simulink model "Sensors"  (R2016b)
settings: Solver=ode45  StartTime=0.0  StopTime=10.0  RelTol=1e-3  EnableMultiTasking=on
undefined symbols (not defined in the file): Amc_flgAirMassFlowOverride, Amc_uSensMaxValid, Amc_uSensMinValid, Bvc_rVoltDivHigh, Bvc_rVoltDivLow, Bvc_uBattMax, Bvc_uBattMin, Cpc_flgPChargeOverride, Ctc_rPullUp_C, Ctc_uSensMaxValid, Ctc_uSensMinValid, Ctc_uSupply, Egc_facEgasMan, Egc_flgEgasOverride, Egc_stEgasFilt, Egc_tiTEgasFilt, Egc_uSensMaxValid, Egc_uSensMinValid, Mpc_uSensMaxValid, Mpc_uSensMinValid, Mtc_rPullUp_C, Mtc_uSensMaxValid, Mtc_uSensMinValid, Mtc_uSupply, Opc_rpmEngMinOilPressure
libraries: simulink x8
(part 2 of 2)

== system Sensors/Sensors_mdl/Opc/G1_Digital_Input_Receive ==
  Data Type Conversion2 : DataTypeConversion  OutMin=0.0  OutMax=1.0  OutDataTypeStr=boolean
  Data Type Conversion3 : DataTypeConversion  OutMin=0.0  OutMax=1.0  OutDataTypeStr=boolean
  FlexECU_DevLib_FcnAPI_Wrapper_SFcn : S-Function  FunctionName=ehooks_medc17flex_devlib_basic_io_fcncall  Parameters=NoInputPorts, NoOutputPorts, InputPortDataTypes, OutputPortDataTypes, CFunctionArgTypes, CFunctionName, ChannelName  SFunctionDeploymentMode=off  EnableBusSupport=off  mask{NoInputPorts=0, NoOutputPorts=2, InputPortDataTypes=, OutputPortDataTypes=uint8,uint8, CFunctionArgTypes=ret,ref, CFunctionName=DevLib_Dio_Get, ChannelName=I_S_DIG13}
      mask prompts: NoInputPorts "Number of input ports"; NoOutputPorts "Number of output ports"; InputPortDataTypes "Input port data types"; OutputPortDataTypes "Output port data types"; CFunctionArgTypes "C function argument types"; CFunctionName "C function name"; ChannelName "Channel (pin) name"
      mask Display: disp('EHOOKS FlexECU\nDevLib Wrapper\nS-Function')
  status : Outport
  stRaw1 : Outport  Port=2
  wires:
  FlexECU_DevLib_FcnAPI_Wrapper_SFcn/2 -> Data Type Conversion2/1
  FlexECU_DevLib_FcnAPI_Wrapper_SFcn/1 -> Data Type Conversion3/1
  Data Type Conversion3/1 -> status/1
  Data Type Conversion2/1 -> stRaw1/1

== system Sensors/Sensors_mdl/Cpc/Cpc_calc/Accumulator ==
  in : Inport
  initValue : Inport  Port=2
  Add : Sum
  MATLAB Function : MATLAB Function  TreatAsAtomicUnit=on
  Switch2 : Switch  Threshold=1
  Unit Delay : UnitDelay  SampleTime=-1
  Out2 : Outport
  wires:
  in/1 -> Add/1, MATLAB Function/1(u)
  Unit Delay/1 -> Add/2
  Switch2/1 -> Out2/1
  initValue/1 -> Switch2/3
  Add/1 -> Switch2/1, Unit Delay/1
  MATLAB Function/1(y) -> Switch2/2

== system Sensors/Sensors_mdl/Cpc/Cpc_calc/Counter ==
  in : Inport
  Add1 : Sum
  Constant1 : Constant  OutDataTypeStr=single
  Constant2 : Constant  Value=0  OutDataTypeStr=single
  MATLAB Function : MATLAB Function  TreatAsAtomicUnit=on
  Switch2 : Switch  Threshold=1
  Unit Delay1 : UnitDelay  SampleTime=-1
  Out1 : Outport
  wires:
  Constant1/1 -> Add1/1
  Unit Delay1/1 -> Add1/2
  Switch2/1 -> Out1/1
  Constant2/1 -> Switch2/3
  Add1/1 -> Switch2/1, Unit Delay1/1
  MATLAB Function/1(y) -> Switch2/2
  in/1 -> MATLAB Function/1(u)

== system Sensors/Sensors_mdl/Cpc/Cpc_get/G1_ADC_Input_Receive ==
  Data Type Conversion2 : DataTypeConversion  OutMin=0.0  OutMax=5.0  OutDataTypeStr=single
  Data Type Conversion3 : DataTypeConversion  OutMin=0.0  OutMax=1.0  OutDataTypeStr=boolean
  FlexECU_DevLib_FcnAPI_Wrapper_SFcn : S-Function  FunctionName=ehooks_medc17flex_devlib_basic_io_fcncall  Parameters=NoInputPorts, NoOutputPorts, InputPortDataTypes, OutputPortDataTypes, CFunctionArgTypes, CFunctionName, ChannelName  SFunctionDeploymentMode=off  EnableBusSupport=off  mask{NoInputPorts=0, NoOutputPorts=2, InputPortDataTypes=, OutputPortDataTypes=uint8,int16, CFunctionArgTypes=ret,ref, CFunctionName=DevLib_Adc_Get, ChannelName=I_A_AN05}
      mask prompts: NoInputPorts "Number of input ports"; NoOutputPorts "Number of output ports"; InputPortDataTypes "Input port data types"; OutputPortDataTypes "Output port data types"; CFunctionArgTypes "C function argument types"; CFunctionName "C function name"; ChannelName "Channel (pin) name"
      mask Display: disp('EHOOKS FlexECU\nDevLib Wrapper\nS-Function')
  Gain : Gain  Gain=5/1023  OutDataTypeStr=Inherit: Same as input
  status : Outport
  uRaw : Outport  Port=2
  wires:
  FlexECU_DevLib_FcnAPI_Wrapper_SFcn/1 -> Data Type Conversion3/1
  FlexECU_DevLib_FcnAPI_Wrapper_SFcn/2 -> Data Type Conversion2/1
  Gain/1 -> uRaw/1
  Data Type Conversion3/1 -> status/1
  Data Type Conversion2/1 -> Gain/1

== system Sensors/Sensors_mdl/Mpc/Mpc_calc/Accumulator ==
  in : Inport
  initValue : Inport  Port=2
  Add : Sum
  MATLAB Function : MATLAB Function  TreatAsAtomicUnit=on
  Switch2 : Switch  Threshold=1
  Unit Delay : UnitDelay  SampleTime=-1
  Out2 : Outport
  wires:
  MATLAB Function/1(y) -> Switch2/2
  Add/1 -> Unit Delay/1, Switch2/1
  initValue/1 -> Switch2/3
  Switch2/1 -> Out2/1
  Unit Delay/1 -> Add/2
  in/1 -> MATLAB Function/1(u), Add/1

== system Sensors/Sensors_mdl/Mpc/Mpc_calc/Counter ==
  in : Inport
  Add1 : Sum
  Constant1 : Constant  OutDataTypeStr=single
  Constant2 : Constant  Value=0  OutDataTypeStr=single
  MATLAB Function : MATLAB Function  TreatAsAtomicUnit=on
  Switch2 : Switch  Threshold=1
  Unit Delay1 : UnitDelay  SampleTime=-1
  Out1 : Outport
  wires:
  in/1 -> MATLAB Function/1(u)
  MATLAB Function/1(y) -> Switch2/2
  Add1/1 -> Unit Delay1/1, Switch2/1
  Constant2/1 -> Switch2/3
  Switch2/1 -> Out1/1
  Unit Delay1/1 -> Add1/2
  Constant1/1 -> Add1/1

== system Sensors/Sensors_mdl/Mpc/Mpc_get/G1_ADC_Input_Receive ==
  Data Type Conversion2 : DataTypeConversion  OutMin=0.0  OutMax=5.0  OutDataTypeStr=single
  Data Type Conversion3 : DataTypeConversion  OutMin=0.0  OutMax=1.0  OutDataTypeStr=boolean
  FlexECU_DevLib_FcnAPI_Wrapper_SFcn : S-Function  FunctionName=ehooks_medc17flex_devlib_basic_io_fcncall  Parameters=NoInputPorts, NoOutputPorts, InputPortDataTypes, OutputPortDataTypes, CFunctionArgTypes, CFunctionName, ChannelName  SFunctionDeploymentMode=off  EnableBusSupport=off  mask{NoInputPorts=0, NoOutputPorts=2, InputPortDataTypes=, OutputPortDataTypes=uint8,int16, CFunctionArgTypes=ret,ref, CFunctionName=DevLib_Adc_Get, ChannelName=I_A_AN05}
      mask prompts: NoInputPorts "Number of input ports"; NoOutputPorts "Number of output ports"; InputPortDataTypes "Input port data types"; OutputPortDataTypes "Output port data types"; CFunctionArgTypes "C function argument types"; CFunctionName "C function name"; ChannelName "Channel (pin) name"
      mask Display: disp('EHOOKS FlexECU\nDevLib Wrapper\nS-Function')
  Gain : Gain  Gain=5/1023  OutDataTypeStr=Inherit: Same as input
  status : Outport
  uRaw : Outport  Port=2
  wires:
  Data Type Conversion2/1 -> Gain/1
  Data Type Conversion3/1 -> status/1
  Gain/1 -> uRaw/1
  FlexECU_DevLib_FcnAPI_Wrapper_SFcn/2 -> Data Type Conversion2/1
  FlexECU_DevLib_FcnAPI_Wrapper_SFcn/1 -> Data Type Conversion3/1

== matlab function Sensors/Sensors_mdl/Egc/LowpassT/MATLAB Function ==
  data: x output; u input; y output
function [x,y]= fcn(u)
% initValue Test
if(u<0)
    y = 0;
else
    y = 1;
end

x = u;

== matlab function Sensors/Sensors_mdl/Egc/LowpassT_Fcn/MATLAB Function ==
  data: u input; y output
function y = fcn(u)
% initValue Test
if(u<0)
    y = 0;
else
    y = 1;
end

== matlab function Sensors/Sensors_mdl/Cpc/Cpc_calc/Accumulator/MATLAB Function ==
  data: u input; y output
function y = fcn(u)
% initValue Test
if(u<=0)
    y = 0;
else
    y = 1;
end

== matlab function Sensors/Sensors_mdl/Cpc/Cpc_calc/Counter/MATLAB Function ==
  data: u input; y output
function y = fcn(u)
% initValue Test
if(u<=0)
    y = 0;
else
    y = 1;
end

== matlab function Sensors/Sensors_mdl/Mpc/Mpc_calc/Accumulator/MATLAB Function ==
  data: u input; y output
function y = fcn(u)
% initValue Test
if(u<=0)
    y = 0;
else
    y = 1;
end

== matlab function Sensors/Sensors_mdl/Mpc/Mpc_calc/Counter/MATLAB Function ==
  data: u input; y output
function y = fcn(u)
% initValue Test
if(u<=0)
    y = 0;
else
    y = 1;
end
